simulink model "navion_demo3"  (Simulink 4.0)
settings: Solver=ode4  StartTime=0.0  StopTime=300  FixedStep=0.05  RelTol=1e-3
libraries: simulink_extras x3, aerosimlib x1
settings Model: LastModifiedBy=mariusn  SaveTime=off  SaveOutput=off  LimitDataPoints=off  UnconnectedInputMsg=none  UnconnectedOutputMsg=none  UnconnectedLineMsg=none  BlockReductionOpt=off

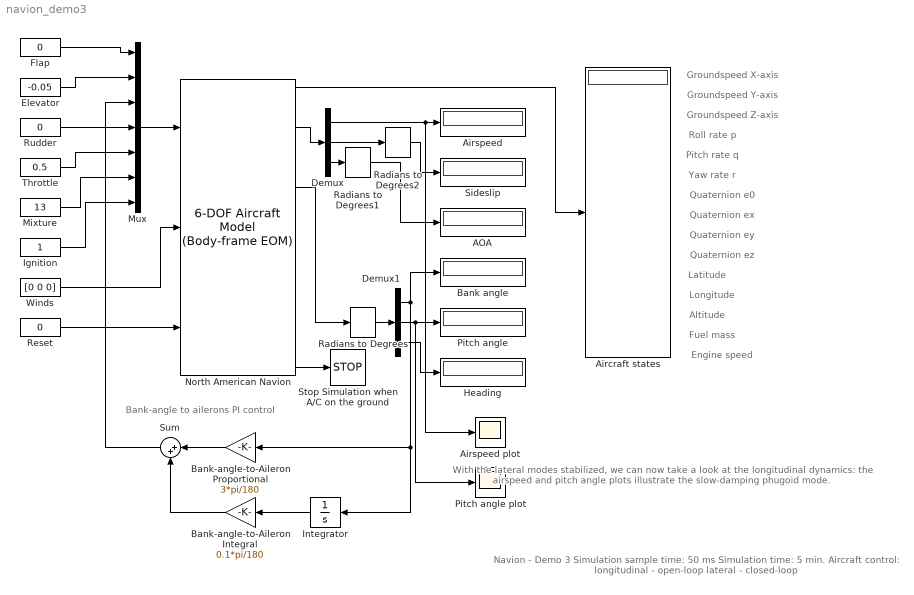
== system navion_demo3 ==
  note: Groundspeed X-axis
  note: Groundspeed Y-axis
  note: Groundspeed Z-axis
  note: Roll rate p
  note: Pitch rate q
  note: Yaw rate r
  note: Quaternion e0
  note: Quaternion ex
  note: Quaternion ey
  note: Quaternion ez
  note: Latitude
  note: Longitude
  note: Altitude
  note: Fuel mass
  note: Engine speed
  note: Navion - Demo 3
      | Simulation sample time: 50 ms
      | Simulation time: 5 min.
      | Aircraft control: longitudinal - open-loop
      |                  lateral - closed-loop
  note: Bank-angle to ailerons PI control
  note: With the lateral modes stabilized, we can now
      | take a look at the longitudinal dynamics: the airspeed
      | and pitch angle plots illustrate the slow-damping
      | phugoid mode.
  AOA : Display
      settings: Format=short
  Aircraft states : Display
      settings: Format=short
  Airspeed : Display
      settings: Format=short
  Airspeed plot : Scope
      settings: TimeRange=300  YMin=40  YMax=52  SaveToWorkspace=off  SaveName=ScopeData  MaxDataPoints=5000
  Bank angle : Display
      settings: Format=short
  Bank-angle-to-Aileron Integral : Gain  Orientation=left  Gain=0.1*pi/180  Multiplication=Element-wise(K.*u)  SaturateOnIntegerOverflow=on
  Bank-angle-to-Aileron Proportional : Gain  Orientation=left  Gain=3*pi/180  Multiplication=Element-wise(K.*u)  SaturateOnIntegerOverflow=on
  Demux : Demux  Outputs=3  BusSelectionMode=off
  Demux1 : Demux  Outputs=3  BusSelectionMode=off
  Elevator : Constant  Value=-0.05
  Flap : Constant  Value=0
  Heading : Display
      settings: Format=short
  Ignition : Constant  Value=1
  Integrator : Integrator  Orientation=left  ExternalReset=none  InitialConditionSource=internal  InitialCondition=0  LimitOutput=off  UpperSaturationLimit=inf  LowerSaturationLimit=-inf  ShowSaturationPort=off  ShowStatePort=off  AbsoluteTolerance=auto
  Mixture : Constant  Value=13
  Mux : Mux  Inputs=7
  North American Navion : aerosimlib/Complete Aircraft/6-DOF Aircraft Model (Body-frame EOM)  aircraftcfg='navioncfg.mat'  VelocitiesIni=[50 0 0]'  RatesIni=[0 0 0]'  QuaternionsIni=[1 0 0 0]'  PositionIni=[45*pi/180 -122*pi/180 1000]'  FuelIni=200  OmegaIni=2400*pi/30  GndAlt=20  wmmfile='C:\Program Files\AeroSim\wmm.cof'  dmy=[09 01 2002]  tsamp=0.05
  Pitch angle : Display
      settings: Format=short
  Pitch angle plot : Scope
      settings: TimeRange=300  YMin=-5  YMax=15  SaveToWorkspace=off  MaxDataPoints=5000
  Radians to Degrees : simulink_extras/Transformations/Radians to Degrees
  Radians to Degrees1 : simulink_extras/Transformations/Radians to Degrees
  Radians to Degrees2 : simulink_extras/Transformations/Radians to Degrees
  Reset : Constant  Value=0
  Rudder : Constant  Value=0
  Sideslip : Display
      settings: Format=short
  Stop Simulation when A/C on the ground : Stop
  Sum : Sum  Orientation=left  Inputs=|++  SaturateOnIntegerOverflow=on
  Throttle : Constant  Value=0.5
  Winds : Constant  Value=[0 0 0]
  wires:
  Reset/1 -> North American Navion/3
  Winds/1 -> North American Navion/2
  North American Navion/1 -> Aircraft states/1
  North American Navion/6 -> Radians to Degrees/1
  North American Navion/3 -> Demux/1
  Demux/3 -> Radians to Degrees1/1
  Demux/2 -> Radians to Degrees2/1
  Demux/1 -> Airspeed/1, Airspeed plot/1
  Radians to Degrees2/1 -> Sideslip/1
  Radians to Degrees1/1 -> AOA/1
  North American Navion/15 -> Stop Simulation when A/C on the ground/1
  Radians to Degrees/1 -> Demux1/1
  Demux1/2 -> Pitch angle/1, Pitch angle plot/1
  Demux1/3 -> Heading/1
  Demux1/1 -> Bank angle/1, Bank-angle-to-Aileron Proportional/1, Integrator/1
  Flap/1 -> Mux/1
  Elevator/1 -> Mux/2
  Rudder/1 -> Mux/4
  Throttle/1 -> Mux/5
  Mixture/1 -> Mux/6
  Ignition/1 -> Mux/7
  Mux/1 -> North American Navion/1
  Bank-angle-to-Aileron Proportional/1 -> Sum/1
  Integrator/1 -> Bank-angle-to-Aileron Integral/1
  Bank-angle-to-Aileron Integral/1 -> Sum/2
  Sum/1 -> Mux/3
